simulink model "sampleModel291original"  (R2021b)
settings: Solver=VariableStepAuto  StartTime=0.0  StopTime=10.0  RelTol=1e-3
libraries: simulink x1
settings Model: Creator=user  LastModifiedBy=cemery

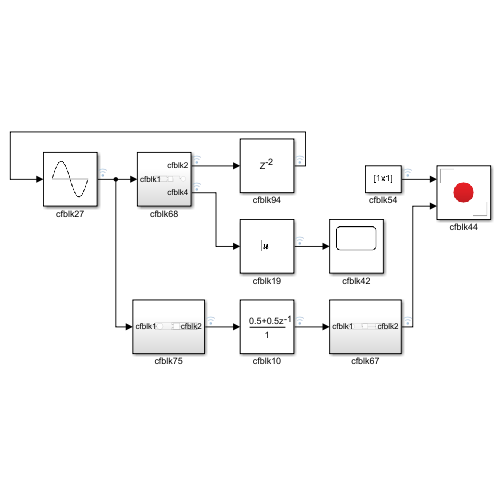
[thumbnail: Simulink's stored preview of the top-level diagram]
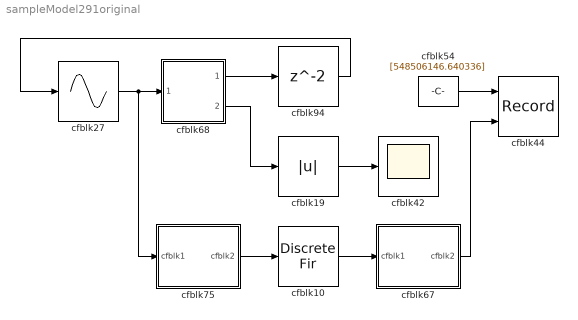
== system sampleModel291original ==
  cfblk10 : DiscreteFir  SampleTime=1
  cfblk19 : Abs
  cfblk27 : Sin  TimeSource=Use external signal  SampleTime=0
  cfblk42 : Scope
  cfblk44 : Record  FileSettingsInternal="{\"entries\":[{\"content\":{\"excelSettings\":{\"content\":{},\"type\":\"Streamout.ExcelSettings\"}},\"type\":\"Streamout.FileSettingStorage\",\"uuid\":\"51942df6-16a4-4685-b70d-2ae4707f6288\"}],\"packageUris\":[\"http://schema.mathworks.com/mf0/streamout_blocks/R2020a\"],\"version\":\"1.0\"}"  Layout=[1 1]  SignalsInternal="{\"entries\":[{\"content\":{\"signals\":[{\"content\":{\"blockPath\":[\"sampleModel291original/cfblk44\"],\"channel\":[],\"dimensions\":[1],\"domain\":\"sampleModel291original/cfblk44\",\"lineColor\":\"#d95319\",\"plots\":[],\"port\":1,\"sid\":[],\"signalID\":107777,\"signalName\":\"cfblk54\"},\"type\":\"RecordBlkView.Signal\",\"uuid\":\"0372f152-a334-46d1-ac6f-9eb17b93906c\"},{\"content\":{\"blockPath\":[\"sampleModel291original/cfblk44\"],\"channel\":[],\"dimensions\":[1],\"domain\":\"sampleModel291original/cfblk44\",\"lineColor\":\"#edb120\",\"plots\":[],\"port\":2,\"sid\":[],\"signalID\":107780,\"signalName\":\"cfblk67\"},\"type\":\"RecordBlkView.Signal\",\"uuid\":\"e36bc5e1-ad04-4298-b1a9-7dd0088d1cb9\"}]},\"type\":\"RecordBlkView.InputSignals\",\"uuid\":\"1dcd026d-489b-4088-b2ee-b02f56987c5d\"}],\"packageUris\":[\"http://schema.mathworks.com/mf0/streamout_blocks/R2020a\"],\"version\":\"1.0\"}"  VisualizationBindings="{\"xyplotplugin\":{\"info\":[{\"series\":[],\"subplotID\":1}]}}"  CompatibilityTag=XY
  cfblk54 : Constant  Value=[548506146.640336]  SampleTime=1
  cfblk67 : Subsystem
  cfblk68 : Subsystem
  cfblk75 : Subsystem
  cfblk94 : Delay  SampleTime=1
  wires:
  cfblk54/1 -> cfblk44/1
  cfblk67/1(cfblk2) -> cfblk44/2
  cfblk19/1 -> cfblk42/1
  cfblk68/1(cfblk2) -> cfblk94/1
  cfblk68/2(cfblk4) -> cfblk19/1
  cfblk94/1 -> cfblk27/1
  cfblk75/1(cfblk2) -> cfblk10/1
  cfblk10/1 -> cfblk67/1(cfblk1)
  cfblk27/1 -> cfblk68/1(cfblk1), cfblk75/1(cfblk1)

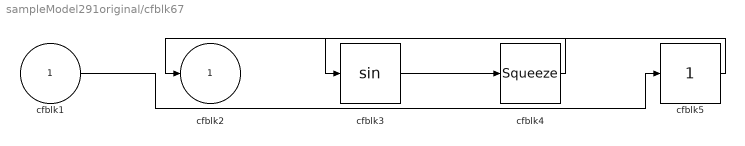
== system sampleModel291original/cfblk67 ==
  cfblk1 : Inport
  cfblk3 : Trigonometry
  cfblk4 : Squeeze
  cfblk5 : simulink/Math Operations/Slider Gain  gain=1  low=0  high=2
  cfblk2 : Outport
  wires:
  cfblk4/1 -> cfblk2/1
  cfblk1/1 -> cfblk5/1
  cfblk3/1 -> cfblk4/1
  cfblk5/1 -> cfblk3/1

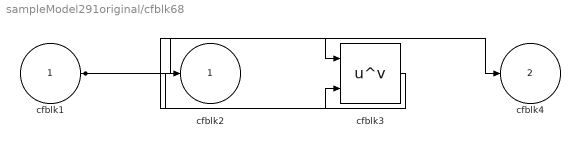
== system sampleModel291original/cfblk68 ==
  cfblk1 : Inport
  cfblk3 : Math  Operator=pow  SaturateOnIntegerOverflow=on
  cfblk2 : Outport
  cfblk4 : Outport  Port=2
  wires:
  cfblk1/1 -> cfblk4/1, cfblk3/1, cfblk3/2
  cfblk3/1 -> cfblk2/1

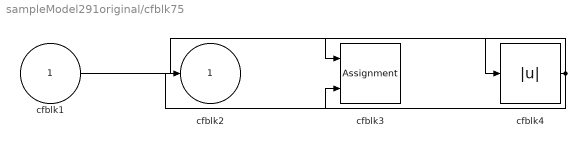
== system sampleModel291original/cfblk75 ==
  cfblk1 : Inport
  cfblk3 : Assignment  DiagnosticForDimensions=Warning  IndexOptions=Index vector (dialog)  Indices=1  OutputSizes=1
  cfblk4 : Abs
  cfblk2 : Outport
  wires:
  cfblk1/1 -> cfblk4/1
  cfblk4/1 -> cfblk2/1, cfblk3/1, cfblk3/2
